simulink model "VPC_onlineGP_triggerTime"  (Simulink 10.3)
settings: Solver=VariableStepAuto  StartTime=0.0  StopTime=50  FixedStep=0.001  RelTol=1e-3
model workspace (MAT data in the model file):
  lambda = 0.0016
  po : num (value not decoded)
undefined symbols (not defined in the file): mergepose, Pinhole
libraries: simlib_vpc_basic x9, simlib_vpc_coremath x7, simlib_vpc_gp x2
settings Model: Creator=marco  LastModifiedBy=marco  MultithreadedSim=on
settings DataIOCC: SaveFormat=Dataset  SignalLoggingSaveFormat=Dataset  ReturnWorkspaceOutputs=on
settings OptimizationCC: ExpressionDepthLimit=128  LifeSpan=auto
settings DebuggingCC: AlgebraicLoopMsg=none  UnderspecifiedInitializationDetection=Simplified  MergeDetectMultiDrivingBlocksExec=error  FcnCallInpInsideContextMsg=error  StateNameClashWarn=none  SFUnexpectedBacktrackingDiag=error  SFNoUnconditionalDefaultTransitionDiag=error  SFExecutionAtInitializationDiag=warning  ArithmeticOperatorsInVariantConditions=error
settings HardwareCC: ProdBitPerPointer=64  ProdBitPerSizeT=64  ProdBitPerPtrDiffT=64  ProdLargestAtomicFloat=Float  ProdIntDivRoundTo=Zero  ProdEndianess=LittleEndian  ProdWordSize=64  ProdHWDeviceType=Intel->x86-64 (Windows64)
settings ModelReferenceCC: PropagateSignalLabelsOutOfModel=on
settings SFSimCC: SimUseLocalCustomCode=on  CustomCodeUndefinedFunction=FilterOut
settings RTWCC: RTWUseLocalCustomCode=on  Toolchain=Clang v3.1 | gmake (64-bit Mac)
settings CodeAppCC: StateflowObjectComments=off
settings GRTTargetCC: TargetLangStandard=C99 (ISO)  CombineOutputUpdateFcns=on  GRTInterface=off
settings ConfigComp: CovMetricSettings=dwe  CovSaveCumulativeToWorkspaceVar=off  CovSaveSingleToWorkspaceVar=off  CovExternalEMLEnable=on

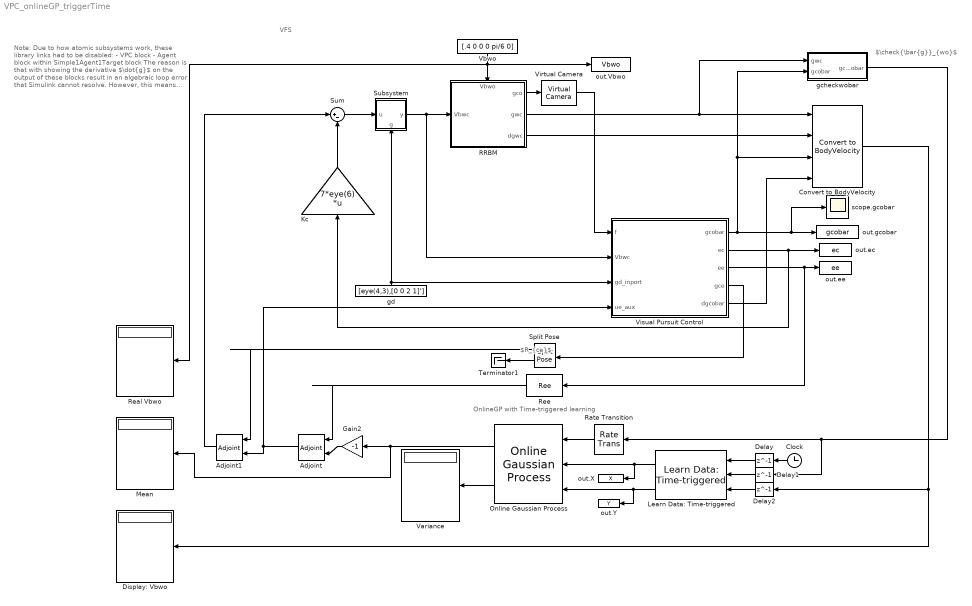
== system VPC_onlineGP_triggerTime ==
  note: VFS
  note: $\check{\bar{g}}_{wo}$
  note: $R_{ce}$
  note: OnlineGP with Time-triggered learning
  note: Note:
      |
      | Due to how atomic subsystems work, these library links had to be disabled:
      | - VPC block
      | - Agent block within Simple1Agent1Target block
      |
      | The reason is that with showing the derivative $\dot{g}$ on the output of these blocks result in an algebraic loop error that Simulink cannot resolve.
      |
      | However, this means that these blocks in this Simulink file are unique and do NOT belong to the library. Please note that changes in the library for these blocks therefore do not affect this Simulink file, and changes have to be made manually!
  Adjoint : simlib_vpc_basic/Adjoint  adjointtype=orientation
      settings: SourceProductName=VPC Library
  Adjoint1 : simlib_vpc_basic/Adjoint  adjointtype=orientation
      settings: SourceProductName=VPC Library
  Clock : Clock
  Convert to BodyVelocity : simlib_vpc_coremath/Convert to BodyVelocity
      settings: SourceProductName=VPC Library
  Delay : Delay  DelayLength=1
  Delay1 : Delay  DelayLength=1  InitialCondition=zeros(6,1)
  Delay2 : Delay  DelayLength=1  InitialCondition=zeros(6,1)
  Display: Vbwo : Display
  Gain2 : Gain  Gain=-1
  Kc : Gain  Gain=7*eye(6)  Multiplication=Matrix(K*u) (u vector)
  Learn Data: Time-triggered : simlib_vpc_gp/Learn Data: Time-triggered  ts=0.01  T=1  M=10  forget_type=oldest
      settings: SourceProductName=VPC Library
  Mean : Display
  Online Gaussian Process : simlib_vpc_gp/Online Gaussian Process  sn_source=internal  sn=1e-2.*ones(6,1)  kernel=Squared Exponential ARD  hyp_source=internal  hyp=[5811173401.07743,21588555449944.6,1,8110042.13413100,7904.61094638263,7904.61094640294,0.200026025926779;60.7489924638542,524.808810512054,1,1.61563170712922,1.71239559901261,1.71239559901241,5.61320776710465e-12;1489.26961783243,49.4500876144320,1,0.324984946298690,0.226613543570055,0.226613543570214,1.82535781762732e-12;0.155449650516185,65.1816809298117,1,38.3822907611281,127.663031081991,127.663031082079,1.99651276292628e-06;128404403992.719,7471024903.20162,1,84140203.5908082,50182603.3525114,50182603.3525587,0.523611111558223;37.3372791443734,0.609451645130079,1,112.088235919108,638.746459440934,638.746459442022,3.48460802714492e-08]
      settings: SourceProductName=VPC Library
  RRBM : Subsystem
      settings: PortSchema="{\"entries\":[{\"content\":{\"sides\":[{\"content\":{\"connectorIds\":[\"In1\"]},\"type\":\"ConnectorPlacement.EquallySpacedRectSide\",\"uuid\":\"ce1006a6-ff18-4db7-ad69-3a60144a672f\"},{\"content\":{\"connectorIds\":[\"Out1\",\"Out2\",\"Out3\"],\"side\":\"RIGHT\"},\"type\":\"ConnectorPlacement.EquallySpacedRectSide\",\"uuid\":\"9f6b7cf2-eb23-4db0-862a-f9244538bf77\"},{\"content\":{\"connectorIds\":[\"In2\"],\"side\":\"TOP\"},\"type\":\"ConnectorPlacement.EquallySpacedRectSide\",\"uuid\":\"e4abfdaf-0145-4439-9abb-46234dad4713\"},{\"content\":{\"connectorIds\":[],\"side\":\"HIDDEN\"},\"type\":\"ConnectorPlacement.EquallySpacedRectSide\",\"uuid\":\"77f0040d-d5e2-4b47-95e1-996605172696\"}]},\"type\":\"ConnectorPlacement.EquallySpacedConnector\",\"uuid\":\"a30e6cf8-5cfd-45cc-9c7f-0b16cc268ba1\"}],\"packageUris\":[\"http://schema.mathworks.com/mf0/Connector/R2020b\"],\"version\":\"1.0\"}"
      mask Display:
      | % Glitch in Matlab: If you define a line whose starting point and end point
      | % is equal, then the entire mask block is plotted in bold
      | plot([0,0],[0,0])
      | 
      | % Draw Box
      | plot([0,1,1,0,0],[0,0,1,1,0])
      | 
      | % Write label
      | fprintf('1 Agent\n1 Target','texmode','on')
      | 
      | % Label ports
      | port_label('input',1,'V^{b}_{wc}','texmode','on')
      | port_label('input',2,'V^{b}_{wo}','texmode','on')
      | port_label('output',1,'g_{co}','texmode','on')
      | port_label('output',2,'g_{wc}','texmode','on')
      | port_label('output',3,'dg_{wc}','texmode','on')
  Rate Transition : RateTransition  OutPortSampleTime=0.01
  Real Vbwo : Display
  Ree : simlib_vpc_coremath/Ree
      settings: SourceProductName=VPC Library
  Split Pose : simlib_vpc_coremath/Split Pose
      settings: SourceProductName=VPC Library
  Subsystem : Subsystem
      settings: PortSchema="{\"entries\":[{\"content\":{\"sides\":[{\"content\":{\"connectorIds\":[\"In1\"]},\"type\":\"ConnectorPlacement.EquallySpacedRectSide\",\"uuid\":\"72e68008-5c4a-43a9-a560-64c6a31a0c08\"},{\"content\":{\"connectorIds\":[\"Out1\"],\"side\":\"RIGHT\"},\"type\":\"ConnectorPlacement.EquallySpacedRectSide\",\"uuid\":\"da07f5ff-2b2c-4c55-a2f2-34e133777503\"},{\"content\":{\"connectorIds\":[],\"side\":\"TOP\"},\"type\":\"ConnectorPlacement.EquallySpacedRectSide\",\"uuid\":\"6d174428-4364-4e89-aba7-4e9864808ab5\"},{\"content\":{\"connectorIds\":[\"In2\"],\"side\":\"BOTTOM\"},\"type\":\"ConnectorPlacement.EquallySpacedRectSide\",\"uuid\":\"f9633104-9c11-4d21-90a7-e0f886d9e92d\"},{\"content\":{\"connectorIds\":[],\"side\":\"HIDDEN\"},\"type\":\"ConnectorPlacement.EquallySpacedRectSide\",\"uuid\":\"662f08ae-9279-4a4f-85ea-81d97ead27d9\"}]},\"type\":\"ConnectorPlacement.EquallySpacedConnector\",\"uuid\":\"f3cd156c-cccd-47c6-b81c-6113f78efd58\"}],\"packageUris\":[\"http://schema.mathworks.com/mf0/Connector/R2020b\"],\"version\":\"1.0\"}"
      mask Display:
      | % Glitch in Matlab: If you define a line whose starting point and end point
      | % is equal, then the entire mask block is plotted in bold
      | plot([0,0],[0,0])
      | 
      | % Draw box
      | indent = 0.3;
      | ang=[0:0.2:pi/2, pi/2];
      | plot([0,1-indent],[0,0])
      | xp=indent*sin(ang)+1-indent;
      | yp=indent-indent*cos(ang);
      | plot(xp,yp);
      | plot([1,1,indent],[indent,1,1])
      | xp=indent-indent*sin(ang);
      | yp=1-indent+indent*cos(ang);
      | plot(xp,yp);
      | plot([0,0],[1-indent,0])
      | 
      | % Write label & ports
      | disp('-Ad_{(g_d)}','texmode','on')
      | text(0.5,0.2,'\fontsize{7}g_d','texmode','on')
  Sum : Sum  Inputs=|+-
  Terminator1 : Terminator
  Variance : Display
  Vbwo : Constant  Value=[.4 0 0 0 pi/6 0]
  Virtual Camera : simlib_vpc_basic/Virtual Camera  camtype=Pinhole  po=po  lambda=lambda
      settings: SourceProductName=VPC Library
  Visual Pursuit Control : Subsystem  mask(Visual Pursuit Control [V1]){gd_source=external, gd_value=[eye(4,3),ones(4,1)], show_ee=on, show_e=off, show_nu=off, show_dgcobar=on, show_gce=on, gcobar0=[eye(4,3), ones(4,1)], Ke_source=internal, Ke=15*eye(6), show_ue_aux=on, projection=on, camtype=Pinhole, fo=po, lambda=lambda}
      mask prompts: gd_source "Desired pose source:"; gd_value "Desired pose"; show_ee "Show estimation error"; show_e "Show total error"; show_nu "Show nu"; show_dgcobar "Show estimation derivative"; show_gce "Show gce"; gcobar0 "Initial estimate gco_bar(0):"; Ke_source "Observer gain source:"; Ke "Observer gain Ke"; show_ue_aux "Show feed-forward ue input"; projection "Use projection"; camtype "Camera type"; fo "Feature point position coordinates (fixed in object frame Σo) [m]"; lambda "Camera focal length λ [m]"
      mask help:
      | Visual Pursuit Control block.
      | Implements the visual pursuit control scheme by incorporating the visual motion observer in a control scenario.
      | Check parameters carefully.
      mask init:
      | % Switch gd: external <-> internal
      | port_number = 3;
      | switch gd_source
      |     case 1 % Make internal
      |         % Delete block & lines
      |         gd = find_system(gcb,'SearchDepth','1','LookUnderMasks','on',...
      |             'FollowLinks','on','Name','gd_inport');
      |         try; delete_line(gcb,'gd_inport/1','Relative Pose/1'); end;
      |         try; delete_block(gd); end;
      | 
      |         % Add block & lines
      |         try; add_block('built-in/Constant',[gcb,'/Desired Pose'],'Value','gd_value','Position',[190 -291 285 -269]); end;
      |         try; add_line(gcb,'Desired Pose/1','Relative Pose/1','autorouting','smart'); end;
      |     case 2 % Make external
      |         % Delete block & lines
      |         gd = find_system(gcb,'SearchDepth','1','LookUnderMasks','on',...
      |             'FollowLinks','on','Name','Desired Pose');
      |         try; delete_line(gcb,'Desired Pose/1','Relative Pose/1'); end;
      |         try; delete_block(gd); end;
      | 
      |         % Add block & lines
      |         try; add_block('built-in/Inport',[gcb,'/gd_inport'],'Port',num2str(port_number),'Position',[220 -287 250 -273]); end;
      |         port_number = port_number + 1;
      |         try; add_line(gcb,'gd_inport/1','Relative Pose/1','autorouting','smart'); end;
      | end
      | 
      | % Switch Ke: external <-> internal
      | switch Ke_source
      |     case 1 % Make internal
      |         % Delete block & lines
      |         Ke_inport = find_system(gcb,'SearchDepth','1','LookUnderMasks','on',...
      |             'FollowLinks','on','Name','Ke_inport');
      |         Ke_mult = find_system(gcb,'SearchDepth','1','LookUnderMasks','on',...
      |             'FollowLinks','on','Name','Ke_mult');
      |         try; delete_line(gcb,'Demux/2','Ke_mult/2'); end;
      |         try; delete_line(gcb,'Ke_inport/1','Ke_mult/1'); end;
      |         try; delete_line(gcb,'Ke_mult/1','Gain/1'); end;
      |         try; delete_block(Ke_mult); end;
      |         try; delete_block(Ke_inport); end;
      | 
      |         % Add block & lines
      |         try; add_block('built-in/Gain',[gcb,'/Ke_gain'],'Gain','Ke','Multiplication','Matrix(K*u) (u vector)','Position',[175 -48 250 28],'Orientation','left'); end;
      |         try; add_line(gcb,'Demux/2','Ke_gain/1','autorouting','smart'); end;
      |         try; add_line(gcb,'Ke_gain/1','Gain/1','autorouting','smart'); end;
      |     case 2 % Make external
      |         % Delete block & lines
      |         Ke_gain = find_system(gcb,'SearchDepth','1','LookUnderMasks','on',...
      |             'FollowLinks','on','Name','Ke_gain');
      |         try; delete_line(gcb,'Demux/2','Ke_gain/1'); end;
      |         try; delete_line(gcb,'Ke_gain/1','Gain/1'); end;
      |         try; delete_block(Ke_gain); end;
      | 
      |         % Add block & lines
      |         try; add_block('built-in/Inport',[gcb,'/Ke_inport'],'Position',[255 -42 285 -28],'Port',num2str(port_number),'Orientation','left'); end;
      |         port_number = port_number + 1;
      |         try; add_block('built-in/Product',[gcb,'/Ke_mult'],'Multiplication','Matrix(*)','Position',[160 -50 210 5],'Orientation','left'); end;
      |         try; add_line(gcb,'Ke_inport/1','Ke_mult/1','autorouting','smart'); end;
      |         try; add_line(gcb,'Demux/2','Ke_mult/2','autorouting','smart'); end;
      |         try; add_line(gcb,'Ke_mult/1','Gain/1','autorouting','smart'); end;
      | end
      | 
      | % Show / Hide: ue_aux
      | if show_ue_aux % Show input
      |     % Delete block & lines
      |     try; delete_line(gcb,'Gain/1','Gain_ue/1'); end;
      | 
      |     % Add block & lines
      |     try; add_block('built-in/Inport',[gcb,'/ue_aux'],'Port',num2str(port_number),'Position',[-150 -132 -120 -118]); end;
      |     try; add_block('built-in/sum',[gcb,'/sum_ue'],'IconShape','round','Position',[-90 -135 -70 -115],'Inputs','|++'); end;
      |     try; add_line(gcb,'ue_aux/1','sum_ue/1','autorouting','smart'); end;
      |     try; add_line(gcb,'Gain/1','sum_ue/2','autorouting','smart'); end;
      |     try; add_line(gcb,'sum_ue/1','Gain_ue/1','autorouting','smart'); end;
      | else % Hide input
      |     % Delete block & lines
      |     ue = find_system(gcb,'SearchDepth','1','LookUnderMasks','on',...
      |         'FollowLinks','on','Name','ue_aux');
      |     sumblock = find_system(gcb,'SearchDepth','1','LookUnderMasks','on',...
      |         'FollowLinks','on','Name','sum_ue');
      |     try; delete_line(gcb,'ue_aux/1','sum_ue/1'); end;
      |     try; delete_line(gcb,'Gain/1','sum_ue/2'); end;
      |     try; delete_line(gcb,'sum_ue/1','Gain_ue/1'); end;
      |     try; delete_block(ue); end;
      |     try; delete_block(sumblock); end;
      | 
      |     % Add block & lines
      |     try; add_line(gcb,'Gain/1','Gain_ue/1','autorouting','smart'); end;
      | end
      | 
      | 
      | %%%%%%%%%%%%%%%%%%
      | %% Outputs
      | %%%%%%%%%%%%%%%%%%
      | 
      | % Show / Hide: ee
      | port_number = 3;
      | if show_ee % Show output
      |     % Add block & lines
      |     try; add_block('built-in/Outport',[gcb,'/ee'],'Port',num2str(port_number),'Position',[515 -122 545 -108]); end;
      |     port_number = port_number + 1;
      |     try; add_line(gcb,'Image Jacobian/1','ee/1','autorouting','smart'); end;
      | else % Hide output
      |     % Delete block & lines
      |     ee = find_system(gcb,'SearchDepth','1','LookUnderMasks','on',...
      |         'FollowLinks','on','Name','ee');
      |     try; delete_line(gcb,'Image Jacobian/1','ee/1'); end;
      |     try; delete_block(ee); end;
      | end
      | 
      | % Show / Hide: e
      | if show_e % Show output
      |     % Add block & lines
      |     try; add_block('built-in/Outport',[gcb,'/e'],'Port',num2str(port_number),'Position',[660 -177 690 -163]); end;
      |     port_number = port_number + 1;
      |     try; add_line(gcb,'Vector Concatenate/1','e/1','autorouting','smart'); end;
      | else % Hide output
      |     % Delete block & lines
      |     e = find_system(gcb,'SearchDepth','1','LookUnderMasks','on',...
      |         'FollowLinks','on','Name','e');
      |     try; delete_line(gcb,'Vector Concatenate/1','e/1'); end;
      |     try; delete_block(e); end;
      | end
      | 
      | % Show / Hide: nu
      | if show_nu % Show output
      |     % Add block & lines
      |     try; add_block('built-in/Outport',[gcb,'/nu'],'Port',num2str(port_number),'Position',[860 -242 890 -228]); end;
      |     port_number = port_number + 1;
      |     try; add_line(gcb,'Matrix Multiply/1','nu/1','autorouting','smart'); end;
      | else % Hide output
      |     % Delete block & lines
      |     nu = find_system(gcb,'SearchDepth','1','LookUnderMasks','on',...
      |         'FollowLinks','on','Name','nu');
      |     try; delete_line(gcb,'Matrix Multiply/1','nu/1'); end;
      |     try; delete_block(nu); end;
      | end
      | 
      | % Show / Hide: gce
      | if show_gce % Show output
      |     % Add block & lines
      |     try; add_block('built-in/Outport',[gcb,'/gce'],'Port',num2str(port_number),'Position',[515 -332 545 -318]); end;
      |     port_number = port_number + 1;
      |     try; add_line(gcb,'Relative Pose/1','gce/1','autorouting','smart'); end;
      | else % Hide output
      |     % Delete block & lines
      |     gce = find_system(gcb,'SearchDepth','1','LookUnderMasks','on',...
      |         'FollowLinks','on','Name','gce');
      |     try; delete_line(gcb,'Relative Pose/1','gce/1'); end;
      |     try; delete_block(gce); end;
      | end
      | 
      | % Show / Hide: dgcobar
      | if show_dgcobar % Show output
      |     % Pass argument to rrbm block
      |     set_param([gcb,'/RRBM'],'show_dgco','on')
      |     % Add block & lines
      |     try; add_block('built-in/Outport',[gcb,'/dgcobar'],'Port',num2str(port_number),'Position',[225 -77 255 -63]); end;
      |     try; add_line(gcb,'RRBM/2','dgcobar/1','autorouting','smart'); end;
      | else
      |     % Delete block & lines
      |     dgcobarblock = find_system(gcb,'SearchDepth','1','LookUnderMasks','on',...
      |         'FollowLinks','on','Name','dgcobar');
      |     try; delete_line(gcb,'RRBM/2','dgcobar/1'); end;
      |     try; delete_block(dgcobarblock); end;
      |     % Pass argument to rrbm block
      |     set_param([gcb,'/RRBM'],'show_dgco','off')
      | end
      settings: MinAlgLoopOccurrences=on
      mask Help:
      | Refer to:
      | T. Hatanaka, N. Chopra, M. Fujita, and M. W. Spong, <i>Passivity-based Control and Estimation in Networked Robotics</i>, ser. Communications and Control Engineering. Springer, 2015.
      mask TypeOptions gd_source: internal | external
      mask Callback gd_source:
      | gd_source = get_param(gcb,'gd_source');
      | 
      | idx = find(strcmp(get_param(gcb,'MaskNames'),'gd_value'));
      | maskvis = get_param(gcb,'MaskVisibilities');
      | switch gd_source
      |     case 'internal' % Show gd field
      |         maskvis{idx} = 'on';
      |     case 'external' % Hide gd field
      |         maskvis{idx} = 'off';
      | end
      | set_param(gcb,'MaskVisibilities',maskvis);
      mask TypeOptions gcobar0: RRBM/gco0
      mask TypeOptions Ke_source: internal | external
      mask Callback Ke_source:
      | Ke_source = get_param(gcb,'Ke_source');
      | 
      | idx = find(strcmp(get_param(gcb,'MaskNames'),'Ke'));
      | maskvis = get_param(gcb,'MaskVisibilities');
      | switch Ke_source
      |     case 'internal' % Show Ke field
      |         maskvis{idx} = 'on';
      |     case 'external' % Hide Ke field
      |         maskvis{idx} = 'off';
      | end
      | set_param(gcb,'MaskVisibilities',maskvis);
      mask TypeOptions projection: RRBM/projection
      mask TypeOptions camtype: Virtual Camera/camtype
      mask TypeOptions fo: Virtual Camera/po
      mask TypeOptions lambda: Virtual Camera/lambda
      mask Display:
      | % Glitch in Matlab: If you define a line whose starting point and end point
      | % is equal, then the entire mask block is plotted in bold
      | plot([0,0],[0,0])
      | 
      | % Draw Box
      | plot([0,1,1,0,0],[0,0,1,1,0])
      | 
      | % Write label
      | p=get_param(gcb,'Position');
      | size = min(p(3:4)-p(1:2));
      | blkscale = abs((p(3)-p(1)) / (p(4)-p(2)));
      | if abs((p(3)-p(1))) > abs((p(4)-p(2))) % block is horizontal
      |     scale = .8*[1/blkscale 1];
      | else % block is vertical
      |     scale = .8*[1 blkscale];
      | end
      | pos = [1-scale(1) 1-scale(2)]./2;
      | image('ico_vmo.png',[pos scale],'off')
      | disp('VPC','texmode','on')
      | 
      | % Label input ports
      | port_label('input',1,'f','texmode','on')
      | port_label('input',2,'V^{b}_{wc}','texmode','on')
      | port_number = 3;
      | gd_source = get_param(gcb, 'gd_source');
      | if gd_source == "external"
      |     port_label('input',port_number,'g_d','texmode','on')
      |     port_number = port_number + 1;
      | end
      | Ke_source = get_param(gcb, 'Ke_source');
      | if Ke_source == "external"
      |         port_label('input',port_number,'K_e','texmode','on')
      |         port_number = port_number + 1;
      | end
      | show_ue_aux = get_param(gcb, 'show_ue_aux');
      | if show_ue_aux == "on"
      |     port_label('input',port_number,'u_{e,aux}','texmode','on')
      | end
      | 
      | % Label output ports
      | port_label('output',1,'g_{co,bar}','texmode','on')
      | port_label('output',2,'e_{c}','texmode','on')
      | port_number = 3;
      | show_ee = get_param(gcb, 'show_ee');
      | if show_ee == "on"
      |     port_label('output',port_number,'e_{e}','texmode','on')
      |     port_number = port_number + 1;
      | end
      | show_e = get_param(gcb, 'show_e');
      | if show_e == "on"
      |     port_label('output',port_number,'e','texmode','on')
      |     port_number = port_number + 1;
      | end
      | show_nu = get_param(gcb, 'show_nu');
      | if show_nu == "on"
      |     port_label('output',port_number,'\nu','texmode','on')
      |     port_number = port_number + 1;
      | end
      | show_gce = get_param(gcb, 'show_gce');
      | if show_gce == "on"
      |     port_label('output',port_number,'g_{ce}','texmode','on')
      |     port_number = port_number + 1;
      | end
      | show_dgcobar = get_param(gcb, 'show_dgcobar');
      | if show_dgcobar == "on"
      |     port_label('output',port_number,'dg_{co,bar}','texmode','on')
      |     port_number = port_number + 1;
      | end
  gcheckwobar : Subsystem
      mask Display:
      | % Write label
      | % disp('Trans','texmode','on')
      | 
      | % Label ports
      | port_label('input',1,'g_{wc}','texmode','on')
      | port_label('input',2,'g_{co,bar}','texmode','on')
      | port_label('output',1,'g^{\upsilon}_{wo,bar}','texmode','on')
  gd : Constant  Value=[eye(4,3),[0 0 2 1]']
  out.Vbwo : ToWorkspace  VariableName=Vbwo  SaveFormat=Structure With Time  SampleTime=-1
  out.X : ToWorkspace  VariableName=X  SaveFormat=Structure With Time  SampleTime=-1
  out.Y : ToWorkspace  VariableName=Y  SaveFormat=Structure With Time  SampleTime=-1
  out.ec : ToWorkspace  VariableName=ec  SaveFormat=Structure With Time  SampleTime=-1
  out.ee : ToWorkspace  VariableName=ee  SaveFormat=Structure With Time  SampleTime=-1
  out.gcobar : ToWorkspace  VariableName=gcobar  SaveFormat=Structure With Time  SampleTime=-1
  scope.gcobar : Scope
  wires:
  Vbwo/1 -> Real Vbwo/1, out.Vbwo/1, RRBM/2(Vbwo)
  RRBM/1(gco) -> Virtual Camera/1
  Virtual Camera/1 -> Visual Pursuit Control/1(f)
  Visual Pursuit Control/1(gcobar) -> out.gcobar/1, scope.gcobar/1, gcheckwobar/2(gcobar), Convert to BodyVelocity/3
  Visual Pursuit Control/2(ec) -> Kc/1, out.ec/1
  Visual Pursuit Control/3(ee) -> Ree/1, out.ee/1
  Subsystem/1(y) -> RRBM/1(Vbwc), Visual Pursuit Control/2(Vbwc)
  Kc/1 -> Sum/2
  gd/1 -> Subsystem/2(g), Visual Pursuit Control/3(gd_inport)
  Ree/1 -> Adjoint/2
  Adjoint/1 -> Adjoint1/1, Visual Pursuit Control/4(ue_aux)
  RRBM/2(gwc) -> Convert to BodyVelocity/1, gcheckwobar/1(gwc)
  Gain2/1 -> Adjoint/1
  Sum/1 -> Subsystem/1(u)
  Adjoint1/1 -> Sum/1
  Visual Pursuit Control/4(gce) -> Split Pose/1
  Split Pose/1 -> Adjoint1/2
  Split Pose/2 -> Terminator1/1
  RRBM/3(dgwc) -> Convert to BodyVelocity/2
  Visual Pursuit Control/5(dgcobar) -> Convert to BodyVelocity/4
  Learn Data: Time-triggered/1 -> out.X/1, Online Gaussian Process/2
  Delay1/1 -> Learn Data: Time-triggered/2
  gcheckwobar/1(gcheck_wobar) -> Rate Transition/1, Delay1/1
  Rate Transition/1 -> Online Gaussian Process/1
  Convert to BodyVelocity/1 -> Display: Vbwo/1, Delay2/1
  Online Gaussian Process/1 -> Gain2/1, Mean/1
  Online Gaussian Process/2 -> Variance/1
  Clock/1 -> Delay/1
  Delay/1 -> Learn Data: Time-triggered/1
  Learn Data: Time-triggered/2 -> out.Y/1, Online Gaussian Process/3
  Delay2/1 -> Learn Data: Time-triggered/3

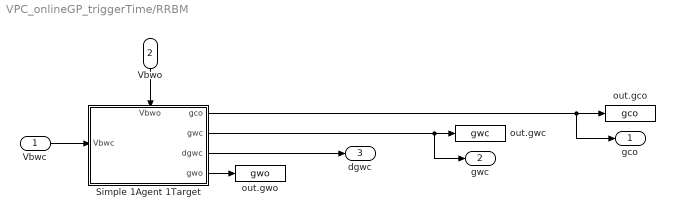
== system VPC_onlineGP_triggerTime/RRBM ==
  Vbwc : Inport
  Vbwo : Inport  Port=2
  Simple 1Agent 1Target : Subsystem  mask(Simple 1Agent 1 Target block [V1]){gwc0=mergepose(rotx(-90),[0; -5; 0]), projectionAgent=on, gwo0=mergepose(rotx(-90),[0.3; 0.1; 0.1]), projectionTarget=on, showgwc=on, showdgwc=on, showgwo=on, showdgwo=off}
      mask prompts: gwc0 "Initial condition gwc(0):"; projectionAgent "Use projection"; gwo0 "Initial condition gwo(0):"; projectionTarget "Use projection"; showgwc "Output gwc"; showdgwc "Output dgwc"; showgwo "Output gwo"; showdgwo "Output dgwo"
      mask help: Implements a simple relative rigid body motion block with one target and one agent.
      mask init:
      | % Blocks
      | gwcblock = find_system(gcb,'LookUnderMasks','on',...
      |     'FollowLinks','on','Name','gwc');
      | dgwcblock = find_system(gcb,'LookUnderMasks','on',...
      |     'FollowLinks','on','Name','dgwc');
      | gwoblock = find_system(gcb,'LookUnderMasks','on',...
      |     'FollowLinks','on','Name','gwo');
      | dgwoblock = find_system(gcb,'LookUnderMasks','on',...
      |     'FollowLinks','on','Name','dgwo');
      | 
      | portnum = 2;
      | 
      | if showgwc % Output gwc
      |     % Add block
      |     try; add_block('built-in/Outport',[gcb,'/gwc'],'Position',[380 128 410 142],'Port',num2str(portnum)); end;
      |     portnum = portnum + 1;
      |     % Connect lines
      |     try; add_line(gcb,'Agent/1','gwc/1','autorouting','smart'); end;
      | else % Hide gwc
      |     % Delete lines
      |     try; delete_line(gcb,'Agent/1','gwc/1'); end;
      |     % Delete block
      |     try; delete_block(gwcblock); end;
      | end
      | 
      | if showdgwc % Output dgwc
      |     % Pass argument to agent block
      |     set_param([gcb,'/Agent'],'show_dg','on')
      |     % Add block
      |     try; add_block('built-in/Outport',[gcb,'/dgwc'],'Position',[200 148 230 162],'Port',num2str(portnum)); end;
      |     portnum = portnum + 1;
      |     % Connect lines
      |     try; add_line(gcb,'Agent/2','dgwc/1','autorouting','smart'); end;
      | else % Hide dgwc
      |     % Delete lines
      |     try; delete_line(gcb,'Agent/2','dgwc/1'); end;
      |     % Delete block
      |     try; delete_block(dgwcblock); end;
      |     % Pass argument to agent block
      |     set_param([gcb,'/Agent'],'show_dg','off')
      | end
      | 
      | if showgwo % Output gwc
      |     % Add block
      |     try; add_block('built-in/Outport',[gcb,'/gwo'],'Position',[380 48 410 62],'Port',num2str(portnum)); end;
      |     portnum = portnum + 1;
      |     % Connect lines
      |     try; add_line(gcb,'Target/1','gwo/1','autorouting','smart'); end;
      | else % Hide gwc
      |     % Delete lines
      |     try; delete_line(gcb,'Target/1','gwo/1'); end;
      |     % Delete block
      |     try; delete_block(gwoblock); end;
      | end
      | 
      | if showdgwo % Output dgwo
      |     % Pass argument to target block
      |     set_param([gcb,'/Target'],'show_dg','on')
      |     % Add block
      |     try; add_block('built-in/Outport',[gcb,'/dgwo'],'Position',[200 63 230 77],'Port',num2str(portnum)); end;
      |     portnum = portnum + 1;
      |     % Connect lines
      |     try; add_line(gcb,'Target/2','dgwo/1','autorouting','smart'); end;
      | else % Hide dgwo
      |     % Delete lines
      |     try; delete_line(gcb,'Target/2','dgwo/1'); end;
      |     % Delete block
      |     try; delete_block(dgwoblock); end;
      |     % Pass argument to agent block
      |     set_param([gcb,'/Target'],'show_dg','off')
      | end
      settings: MinAlgLoopOccurrences=on  PortSchema="{\"entries\":[{\"content\":{\"sides\":[{\"content\":{\"connectorIds\":[\"In1\"]},\"type\":\"ConnectorPlacement.EquallySpacedRectSide\",\"uuid\":\"51848c78-49bf-4d69-8138-12848c04a52b\"},{\"content\":{\"connectorIds\":[\"Out1\",\"Out2\",\"Out3\",\"Out4\"],\"side\":\"RIGHT\"},\"type\":\"ConnectorPlacement.EquallySpacedRectSide\",\"uuid\":\"a2771237-d1b3-407b-8d53-6a34779e1c0e\"},{\"content\":{\"connectorIds\":[\"In2\"],\"side\":\"TOP\"},\"type\":\"ConnectorPlacement.EquallySpacedRectSide\",\"uuid\":\"c6712b15-7cf3-4a58-80e7-6bd7851abb53\"},{\"content\":{\"connectorIds\":[],\"side\":\"HIDDEN\"},\"type\":\"ConnectorPlacement.EquallySpacedRectSide\",\"uuid\":\"8616ed9a-8306-41f0-bffd-55839930ff42\"}]},\"type\":\"ConnectorPlacement.EquallySpacedConnector\",\"uuid\":\"4f48229c-43f3-4c05-9119-4c52932f0077\"}],\"packageUris\":[\"http://schema.mathworks.com/mf0/Connector/R2020b\"],\"version\":\"1.0\"}"
      mask Help:
      | Refer to:
      | T. Hatanaka, N. Chopra, M. Fujita, and M. W. Spong, <i>Passivity-based Control and Estimation in Networked Robotics</i>, ser. Communications and Control Engineering. Springer, 2015.
      mask TypeOptions gwc0: Agent/g0
      mask TypeOptions projectionAgent: Agent/projection
      mask TypeOptions gwo0: Target/g0
      mask TypeOptions projectionTarget: Target/projection
      mask Display:
      | % Glitch in Matlab: If you define a line whose starting point and end point
      | % is equal, then the entire mask block is plotted in bold
      | plot([0,0],[0,0])
      | 
      | % Draw Box
      | plot([0,1,1,0,0],[0,0,1,1,0])
      | 
      | % Write label
      | fprintf('1 Agent\n1 Target','texmode','on')
      | 
      | % Label ports
      | port_label('input',1,'V^{b}_{wc}','texmode','on')
      | port_label('input',2,'V^{b}_{wo}','texmode','on')
      | port_label('output',1,'g_{co}','texmode','on')
      | 
      | % Label dynamic output ports
      | portnumber = 2;
      | if strcmp(get_param(gcb, 'showgwc'),'on')
      |     port_label('output',portnumber,'g_{wc}','texmode','on')
      |     portnumber = portnumber + 1;
      | end
      | if strcmp(get_param(gcb, 'showdgwc'),'on')
      |     port_label('output',portnumber,'dg_{wc}','texmode','on')
      |     portnumber = portnumber + 1;
      | end
      | if strcmp(get_param(gcb, 'showgwo'),'on')
      |     port_label('output',portnumber,'g_{wo}','texmode','on')
      |     portnumber = portnumber + 1;
      | end
      | if strcmp(get_param(gcb, 'showdgwo'),'on')
      |     port_label('output',portnumber,'dg_{wo}','texmode','on')
      |     portnumber = portnumber + 1;
      | end
  out.gco : ToWorkspace  VariableName=gco  SaveFormat=Structure With Time  SampleTime=-1
  out.gwc : ToWorkspace  VariableName=gwc  SaveFormat=Structure With Time  SampleTime=-1
  out.gwo : ToWorkspace  VariableName=gwo  SaveFormat=Structure With Time  SampleTime=-1
  gco : Outport
  gwc : Outport  Port=2
  dgwc : Outport  Port=3
  wires:
  Vbwo/1 -> Simple 1Agent 1Target/2(Vbwo)
  Vbwc/1 -> Simple 1Agent 1Target/1(Vbwc)
  Simple 1Agent 1Target/2(gwc) -> gwc/1, out.gwc/1
  Simple 1Agent 1Target/4(gwo) -> out.gwo/1
  Simple 1Agent 1Target/1(gco) -> gco/1, out.gco/1
  Simple 1Agent 1Target/3(dgwc) -> dgwc/1

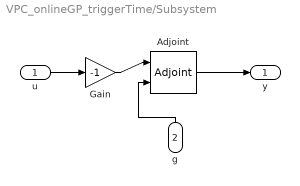
== system VPC_onlineGP_triggerTime/Subsystem ==
  u : Inport
  g : Inport  Port=2
  Adjoint : simlib_vpc_basic/Adjoint  adjointtype=pose
      settings: SourceProductName=VPC Library
  Gain : Gain  Gain=-1
  y : Outport
  wires:
  Adjoint/1 -> y/1
  u/1 -> Gain/1
  g/1 -> Adjoint/2
  Gain/1 -> Adjoint/1

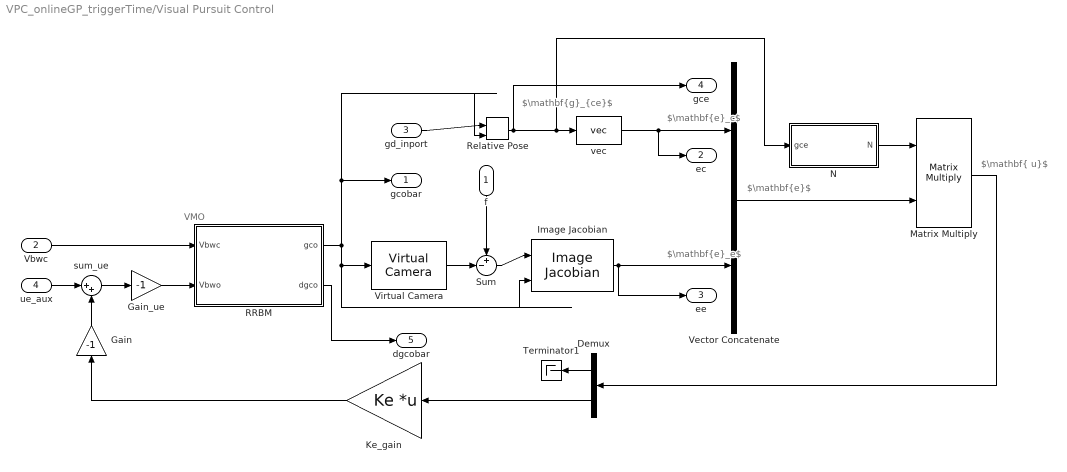
== system VPC_onlineGP_triggerTime/Visual Pursuit Control ==
  note: $\mathbf{\nu}$
  note: $\mathbf{g}_{ce}$
  note: $\mathbf{e}$
  note: $\mathbf{e}_e$
  note: $\mathbf{e}_c$
  note: VMO
  f : Inport
  Vbwc : Inport  Port=2
  gd_inport : Inport  Port=3
  ue_aux : Inport  Port=4
  Demux : Demux  Outputs=2
  Gain : Gain  Gain=-1
  Gain_ue : Gain  Gain=-1
  Image Jacobian : simlib_vpc_basic/Image Jacobian  po=fo  lambda=lambda
      settings: SourceProductName=VPC Library
  Ke_gain : Gain  Gain=Ke  Multiplication=Matrix(K*u) (u vector)
  Matrix Multiply : Product  Multiplication=Matrix(*)
  N : MATLAB Function  TreatAsAtomicUnit=on
  RRBM : Subsystem  mask(Relative Rigid Body Motion Block [V1]){gco0=gcobar0, projection=on, show_dgco=on}
      mask prompts: gco0 "Initial condition gco(0):"; projection "Use projection"; show_dgco "Show dgco"
      mask help: Relative rigid body motion of agent A as it can be observed from agent B.
      mask init:
      | block = find_system(gcb,'LookUnderMasks','on',...
      |     'FollowLinks','on','Name','Projection');
      | 
      | if projection && isempty(block) % Turn on projection
      |     % Delete lines
      |     delete_line(gcb,'Integrator/1','gco/1')
      |     delete_line(gcb,'Integrator/1','rrbm/3')
      |     
      |     % Add block
      |     add_block([bdroot(gcb),'/Projection'],[gcb,'/Projection'],'inputtype','pose');
      |     
      |     % Connect lines
      |     add_line(gcb,'Integrator/1','Projection/1','autorouting','smart')
      |     add_line(gcb,'Projection/1','gco/1','autorouting','smart')
      |     add_line(gcb,'Projection/1','rrbm/3','autorouting','smart')
      | elseif ~projection && ~isempty(block) % Turn off projection
      |     % Delete lines
      |     delete_line(gcb,'Integrator/1','Projection/1')
      |     delete_line(gcb,'Projection/1','gco/1')
      |     delete_line(gcb,'Projection/1','rrbm/3')
      | 
      |     % Delete block
      |     delete_block(block);
      | 
      |     % Connect blocks
      |     add_line(gcb,'Integrator/1','gco/1','autorouting','smart')
      |     add_line(gcb,'Integrator/1','rrbm/3','autorouting','smart')
      | end
      | 
      | % Show dgco output
      | if show_dgco
      |     % Add block & lines
      |     try; add_block('built-in/Outport',[gcb,'/dgco'],'Port','2','Position',[510 193 540 207]); end;
      |     try; add_line(gcb,'rrbm/1','dgco/1','autorouting','smart'); end;
      | else
      |     % Delete block & lines
      |     dgcoblock = find_system(gcb,'SearchDepth','1','LookUnderMasks','on',...
      |         'FollowLinks','on','Name','dgco');
      |     try; delete_line(gcb,'rrbm/1','dgco/1'); end;
      |     try; delete_block(dgcoblock); end;
      | end
      settings: MinAlgLoopOccurrences=on
      mask Help:
      | Refer to:
      | T. Hatanaka, N. Chopra, M. Fujita, and M. W. Spong, <i>Passivity-based Control and Estimation in Networked Robotics</i>, ser. Communications and Control Engineering. Springer, 2015.
      mask TypeOptions gco0: Integrator/InitialCondition
      mask DialogControl show_dgco Tooltip: If on, the internal state derivative of gco will be shown as an output
      mask Display:
      | % Glitch in Matlab: If you define a line whose starting point and end point
      | % is equal, then the entire mask block is plotted in bold
      | plot([0,0],[0,0])
      | 
      | % Draw Box
      | plot([0,1,1,0,0],[0,0,1,1,0])
      | 
      | % Write label
      | fprintf('Relative Rigid\nBody Motion','texmode','on')
      | 
      | % Label ports
      | port_label('input',1,'V^{b}_{wc}','texmode','on')
      | port_label('input',2,'V^{b}_{wo}','texmode','on')
      | port_label('output',1,'g_{co}','texmode','on')
      | if strcmp(get_param(gcb,'show_dgco'),'on')
      |     port_label('output',2,'dg_{co}','texmode','on')
      | end
  Relative Pose : simlib_vpc_coremath/Relative Pose
      settings: SourceProductName=VPC Library
  Sum : Sum  Inputs=+-|
  Terminator1 : Terminator
  Vector Concatenate : Concatenate
  Virtual Camera : simlib_vpc_basic/Virtual Camera  camtype=Pinhole  po=fo  lambda=lambda
      settings: SourceProductName=VPC Library
  sum_ue : Sum  Inputs=|++
  vec : simlib_vpc_coremath/vec
      settings: SourceProductName=VPC Library
  gcobar : Outport
  ec : Outport  Port=2
  ee : Outport  Port=3
  gce : Outport  Port=4
  dgcobar : Outport  Port=5
  wires:
  Ke_gain/1 -> Gain/1
  Demux/2 -> Ke_gain/1
  Demux/1 -> Terminator1/1
  Virtual Camera/1 -> Sum/2
  Gain_ue/1 -> RRBM/2(Vbwo)
  f/1 -> Sum/1
  Sum/1 -> Image Jacobian/1
  Vbwc/1 -> RRBM/1(Vbwc)
  RRBM/1(gco) -> Virtual Camera/1, Image Jacobian/2, gcobar/1, Relative Pose/2
  Image Jacobian/1 -> Vector Concatenate/2, ee/1
  vec/1 -> ec/1, Vector Concatenate/1
  N/1(N) -> Matrix Multiply/1
  Matrix Multiply/1 -> Demux/1
  Vector Concatenate/1 -> Matrix Multiply/2
  Relative Pose/1 -> vec/1, N/1(gce), gce/1
  gd_inport/1 -> Relative Pose/1
  ue_aux/1 -> sum_ue/1
  Gain/1 -> sum_ue/2
  sum_ue/1 -> Gain_ue/1
  RRBM/2(dgco) -> dgcobar/1

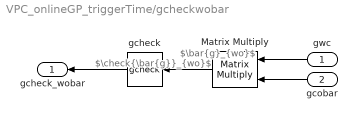
== system VPC_onlineGP_triggerTime/gcheckwobar ==
  note: $\bar{g}_{wo}$
  note: $\check{\bar{g}}_{wo}$
  gwc : Inport
  gcobar : Inport  Port=2
  Matrix Multiply : Product  Multiplication=Matrix(*)
  gcheck : simlib_vpc_coremath/gcheck
      settings: SourceProductName=VPC Library
  gcheck_wobar : Outport
  wires:
  gwc/1 -> Matrix Multiply/1
  gcobar/1 -> Matrix Multiply/2
  gcheck/1 -> gcheck_wobar/1
  Matrix Multiply/1 -> gcheck/1

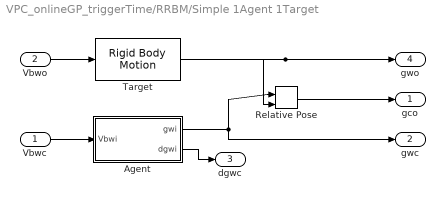
== system VPC_onlineGP_triggerTime/RRBM/Simple 1Agent 1Target ==
  Vbwc : Inport
  Vbwo : Inport  Port=2
  Agent : Subsystem  mask(Rigid Body Motion Block [V1]){rbmtype=agent, agentnumber=1, projection=on, show_dg=on, g0=gwc0}
      mask prompts: rbmtype "Type:"; agentnumber "#"; projection "Use projection"; show_dg "Show derivative dg"; g0 "Initial condition g(0):"
      mask help:
      | Implements a simple (single-integrator-type) rigid body motion model.
      | The RBM type in the parameter pane is just for a better visualization purpose and does not have any effect on the dynamics, but the block mask appearance.
      mask init:
      | block = find_system(gcb,'LookUnderMasks','on',...
      |     'FollowLinks','on','Name','Projection');
      | 
      | if projection && isempty(block) % Turn on projection
      |     % Delete lines
      |     delete_line(gcb,'Integrator/1','gwi/1')
      |     delete_line(gcb,'Integrator/1','rbm/2')
      |     
      |     % Add block
      |     add_block([bdroot(gcb),'/Projection'],[gcb,'/Projection'],'inputtype','pose');
      |     
      |     % Connect lines
      |     add_line(gcb,'Integrator/1','Projection/1','autorouting','smart')
      |     add_line(gcb,'Projection/1','gwi/1','autorouting','smart')
      |     add_line(gcb,'Projection/1','rbm/2','autorouting','smart')
      | elseif ~projection && ~isempty(block) % Turn off projection
      |     % Delete lines
      |     delete_line(gcb,'Integrator/1','Projection/1')
      |     delete_line(gcb,'Projection/1','gwi/1')
      |     delete_line(gcb,'Projection/1','rbm/2')
      | 
      |     % Delete block
      |     delete_block(block);
      | 
      |     % Connect blocks
      |     add_line(gcb,'Integrator/1','gwi/1','autorouting','smart')
      |     add_line(gcb,'Integrator/1','rbm/2','autorouting','smart')
      | end
      | 
      | % Show derivative output dg
      | if show_dg
      |     % Add block & lines
      |     try; add_block('built-in/Outport',[gcb,'/dgwi'],'Port','2','Position',[515 203 545 217]); end;
      |     try; add_line(gcb,'rbm/1','dgwi/1','autorouting','smart'); end;
      | else
      |     % Delete block & lines
      |     dgwiblock = find_system(gcb,'SearchDepth','1','LookUnderMasks','on',...
      |         'FollowLinks','on','Name','dgwi');
      |     try; delete_line(gcb,'rbm/1','dgwi/1'); end;
      |     try; delete_block(dgwiblock); end;
      | end
      settings: MinAlgLoopOccurrences=on
      mask Help:
      | Refer to:
      | T. Hatanaka, N. Chopra, M. Fujita, and M. W. Spong, <i>Passivity-based Control and Estimation in Networked Robotics</i>, ser. Communications and Control Engineering. Springer, 2015.
      mask TypeOptions rbmtype: agent | target
      mask Callback rbmtype:
      | rbmtype = get_param(gcb,'rbmtype');
      | 
      | switch rbmtype
      |     case 'agent'
      |         % Turn on number field
      |         set_param(gcb,'MaskVisibilities',{'on';'on';'on';'on';'on'});
      |     case 'target'
      |         % Turn off number field
      |         set_param(gcb,'MaskVisibilities',{'on';'off';'on';'on';'on'});
      |         % Set number in the invisible field to 0
      |         % set_param(gcb,'agentnumber','0');
      | end
      mask Display:
      | % Glitch in Matlab: If you define a line whose starting point and end point
      | % is equal, then the entire mask block is plotted in bold
      | plot([0,0],[0,0])
      | 
      | % Draw Box
      | plot([0,1,1,0,0],[0,0,1,1,0])
      | 
      | % Write label
      | rbmtype = get_param(gcb, 'rbmtype');
      | switch rbmtype
      |     case 'agent'
      |         agentnumber = get_param(gcb, 'agentnumber');
      |         disp('Agent','texmode','on')
      | 
      |         % Image
      |         p=get_param(gcb,'Position');
      |         size = min(p(3:4)-p(1:2));
      |         blkscale = abs((p(3)-p(1)) / (p(4)-p(2)));
      |         if abs((p(3)-p(1))) > abs((p(4)-p(2))) % block is horizontal
      |             scale = .5*[1/blkscale .6];
      |         else % block is vertical
      |             scale = .5*[1 .6*blkscale];
      |         end
      |         pos = [1-scale(1) 0.1]/2;
      |         image('ico_agent.png',[pos scale],'off')
      |     case 'target'
      |         agentnumber = 0;
      |         disp('Target','texmode','on')
      | 
      |         % Image
      |         p=get_param(gcb,'Position');
      |         size = min(p(3:4)-p(1:2));
      |         blkscale = abs((p(3)-p(1)) / (p(4)-p(2)));
      |         if abs((p(3)-p(1))) > abs((p(4)-p(2))) % block is horizontal
      |             scale = .5*[1/blkscale .6];
      |         else % block is vertical
      |             scale = .5*[1 .6*blkscale];
      |         end
      |         pos = [1-scale(1) 0.1]/2;
      |         image('ico_target.png',[pos scale],'off')
      | end
      | 
      | % Label ports
      | port_label('input',1,['V^{b}_{w' num2str(agentnumber) '}'],'texmode','on')
      | port_label('output',1,['g_{w' num2str(agentnumber) '}'],'texmode','on')
      | if strcmp(get_param(gcb, 'show_dg'),'on')
      |     port_label('output',2,['dg_{w' num2str(agentnumber) '}'],'texmode','on')
      | end
  Relative Pose : simlib_vpc_coremath/Relative Pose
      settings: SourceProductName=VPC Library
  Target : simlib_vpc_basic/Rigid Body Motion  rbmtype=target  agentnumber=1  projection=on  show_dg=off  g0=gwo0
      settings: SourceProductName=VPC Library
  gco : Outport
  gwc : Outport  Port=2
  dgwc : Outport  Port=3
  gwo : Outport  Port=4
  wires:
  Agent/1(gwi) -> gwc/1, Relative Pose/1
  Vbwo/1 -> Target/1
  Target/1 -> gwo/1, Relative Pose/2
  Relative Pose/1 -> gco/1
  Vbwc/1 -> Agent/1(Vbwi)
  Agent/2(dgwi) -> dgwc/1

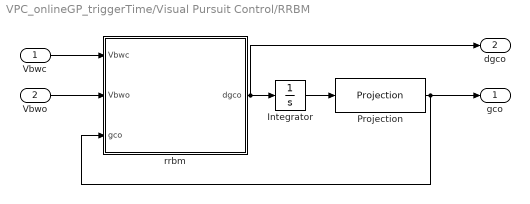
== system VPC_onlineGP_triggerTime/Visual Pursuit Control/RRBM ==
  Vbwc : Inport
  Vbwo : Inport  Port=2
  Integrator : Integrator  InitialCondition=gco0
  Projection : simlib_vpc_basic/Projection  projectiontype=averaging  inputtype=pose
      settings: SourceProductName=VPC Library
  rrbm : MATLAB Function  TreatAsAtomicUnit=on
  gco : Outport
  dgco : Outport  Port=2
  wires:
  Vbwc/1 -> rrbm/1(Vbwc)
  rrbm/1(dgco) -> Integrator/1, dgco/1
  Vbwo/1 -> rrbm/2(Vbwo)
  Integrator/1 -> Projection/1
  Projection/1 -> gco/1, rrbm/3(gco)

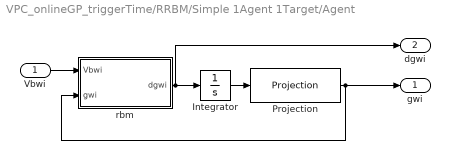
== system VPC_onlineGP_triggerTime/RRBM/Simple 1Agent 1Target/Agent ==
  Vbwi : Inport
  Integrator : Integrator  InitialCondition=g0  ContinuousStateAttributes='pose'
  Projection : simlib_vpc_basic/Projection  projectiontype=averaging  inputtype=pose
      settings: SourceProductName=VPC Library
  rbm : MATLAB Function  TreatAsAtomicUnit=on
  gwi : Outport
  dgwi : Outport  Port=2
  wires:
  Projection/1 -> rbm/2(gwi), gwi/1
  Integrator/1 -> Projection/1
  Vbwi/1 -> rbm/1(Vbwi)
  rbm/1(dgwi) -> Integrator/1, dgwi/1

== matlab function RRBM/Simple 1Agent 1Target/Agent/rbm ==
  data: Vbwi input double size=6; dgwi output double size=[4,4]; gwi input double size=[4,4]
function dgwi = slx_rbm(Vbwi,gwi) %#codegen
% Function Wrapper
%
% Editor:
%   OMAINSKA Marco - Doctoral Student, Cybernetics
%       <marcoomainska@g.ecc.u-tokyo.ac.jp>
% Review:
%   YAMAUCHI Junya - Assistant Professor
%       <junya_yamauchi@ipc.i.u-tokyo.ac.jp>
%
% Property of: Fujita-Yamauchi Lab, University of Tokyo, 2021
% e-mail: marcoomainska@g.ecc.u-tokyo.ac.jp
% Website: https://www.scl.ipc.i.u-tokyo.ac.jp
% March 2021, Last modified: 2021-MAR-08
%
%------------- BEGIN CODE --------------

% "rbm" is a MATLAB function on the MATLAB path
dgwi = rbm(Vbwi, gwi);

%------------- END CODE --------------
end

== matlab function Visual Pursuit Control/RRBM/rrbm ==
  data: Vbwc input double size=6; Vbwo input double size=6; dgco output double size=[4,4]; gco input double size=[4,4]
function dgco = slx_rrbm(Vbwc,Vbwo,gco) %#codegen
% Function Wrapper
%
% Editor:
%   OMAINSKA Marco - Doctoral Student, Cybernetics
%       <marcoomainska@g.ecc.u-tokyo.ac.jp>
% Review:
%   YAMAUCHI Junya - Assistant Professor
%       <junya_yamauchi@ipc.i.u-tokyo.ac.jp>
%
% Property of: Fujita-Yamauchi Lab, University of Tokyo, 2021
% e-mail: marcoomainska@g.ecc.u-tokyo.ac.jp
% Website: https://www.scl.ipc.i.u-tokyo.ac.jp
% March 2021, Last modified: 2021-MAR-08
%
%------------- BEGIN CODE --------------

% "rrbm" is a MATLAB function on the MATLAB path
dgco = rrbm(Vbwc, Vbwo, gco);

%------------- END CODE --------------
end

== matlab function Visual Pursuit Control/N ==
  data: gce input double size=[4,4]; N output double size=[12,12]
function N = slx_NAdj(gce) %#codegen
% Function Wrapper
%
% Editor:
%   OMAINSKA Marco - Doctoral Student, Cybernetics
%       <marcoomainska@g.ecc.u-tokyo.ac.jp>
% Review:
%   YAMAUCHI Junya - Assistant Professor
%       <junya_yamauchi@ipc.i.u-tokyo.ac.jp>
%
% Property of: Fujita-Yamauchi Lab, University of Tokyo, 2021
% e-mail: marcoomainska@g.ecc.u-tokyo.ac.jp
% Website: https://www.scl.ipc.i.u-tokyo.ac.jp
% March 2021, Last modified: 2021-MAR-08
%
%------------- BEGIN CODE --------------

% "NAdj" is a MATLAB function on the MATLAB path
N = NAdj(gce);

%------------- END CODE --------------
end
